simulink model "sampleModel355"  (R2021b)
settings: Solver=VariableStepAuto  StartTime=0.0  StopTime=10.0  RelTol=1e-3
undefined symbols (not defined in the file or in its folder): Newton, Raphson
libraries: simulink x9, slpidlib x1
settings Model: Creator=user  LastModifiedBy=user

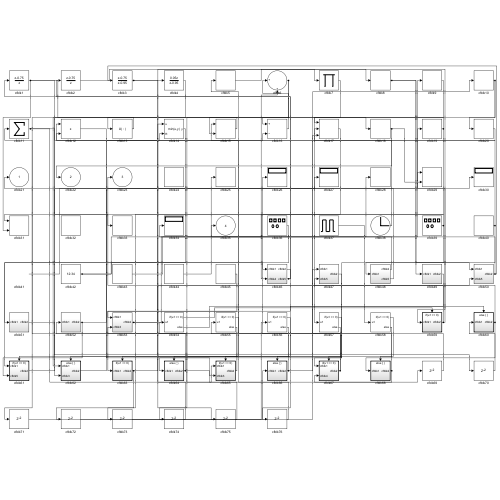
[thumbnail: Simulink's stored preview of the top-level diagram]
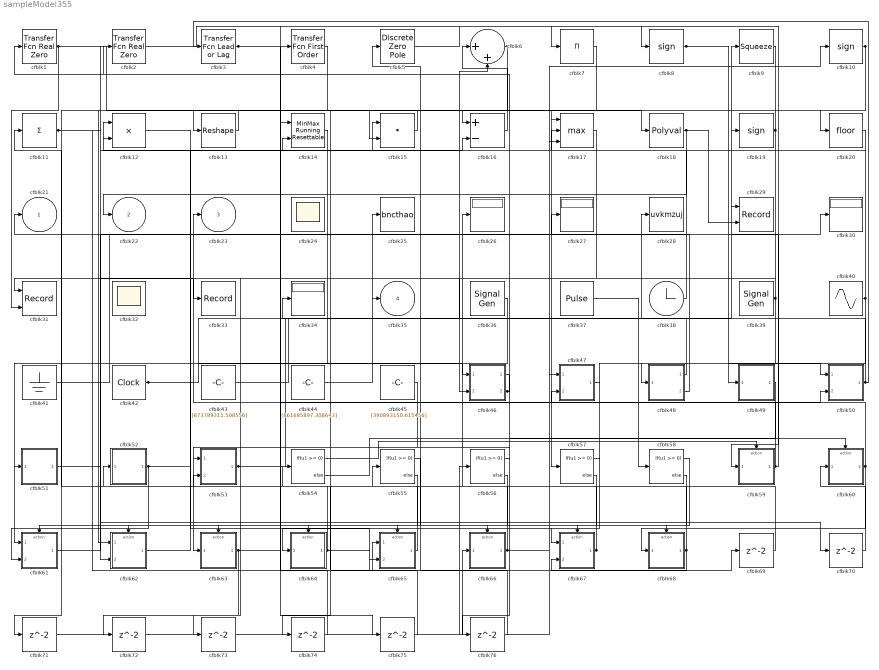
== system sampleModel355 ==
  cfblk1 : simulink/Discrete/Transfer Fcn Real Zero  ZeroZ=0.75  ICPrevInput=0.0  DoSatur=off
      settings: SourceProductBaseCode=SL
  cfblk10 : Signum
  cfblk11 : Sum  Inputs=+
  cfblk12 : Product
  cfblk13 : Reshape
  cfblk14 : simulink/Math Operations/MinMax Running Resettable  Function=min  vinit=0.0
  cfblk15 : DotProduct  InputSameDT=on  OutDataTypeStr=Inherit: Inherit via internal rule
  cfblk16 : Sum  Inputs=+-
  cfblk17 : MinMax  Function=max  Inputs=3
  cfblk18 : Polyval  Coefs=[ +2.081618890e-019, -1.441693666e-014, +4.719686976e-010, -8.536869453e-006, +1.621573104e-001, -8.087801117e+001 ]
  cfblk19 : Signum
  cfblk2 : simulink/Discrete/Transfer Fcn Real Zero  ZeroZ=0.75  ICPrevInput=0.0  DoSatur=off
      settings: SourceProductBaseCode=SL
  cfblk20 : Rounding
  cfblk24 : Scope
      settings: Floating=on
  cfblk25 : ToWorkspace  VariableName=bncthao  SaveFormat=Timeseries  SampleTime=-1
  cfblk{26..27,30,34} (4 alike) : Display
  cfblk28 : ToWorkspace  VariableName=uvkmzuj  SaveFormat=Timeseries  SampleTime=-1
  cfblk29 : Record  FileSettingsInternal="{\"entries\":[{\"content\":{\"excelSettings\":{\"content\":{},\"type\":\"Streamout.ExcelSettings\"}},\"type\":\"Streamout.FileSettingStorage\",\"uuid\":\"8a58f875-e99c-4c1f-ba3d-aacceb243502\"}],\"packageUris\":[\"http://schema.mathworks.com/mf0/streamout_blocks/R2020a\"],\"version\":\"1.0\"}"  Layout=[1 1]  SignalsInternal="{\"entries\":[{\"content\":{\"signals\":[{\"content\":{\"blockPath\":[\"sampleModel355/cfblk29\"],\"channel\":[],\"dimensions\":[1],\"domain\":\"sampleModel355/cfblk29\",\"lineColor\":\"#a2142f\",\"plots\":[1],\"port\":1,\"sid\":[\"\"],\"signalID\":14784,\"signalName\":\"cfblk59\"},\"type\":\"RecordBlkView.Signal\",\"uuid\":\"3281cb25-1353-4514-a61d-ab6e319669d4\"},{\"content\":{\"blockPath\":[\"sampleModel355/cfblk29\"],\"channel\":[],\"dimensions\":[1],\"domain\":\"sampleModel355/cfblk29\",\"lineColor\":\"#139fff\",\"plots\":[1],\"port\":2,\"sid\":[\"\"],\"signalID\":14788,\"signalName\":\"cfblk18\"},\"type\":\"RecordBlkView.Signal\",\"uuid\":\"1768254f-e474-4347-aa62-2856f5bec4c9\"}]},\"type\":\"RecordBlkView.InputSignals\",\"uuid\":\"2a2635e2-e26a-4ce4-9f08-0e49d7d24d48\"}],\"packageUris\":[\"http://schema.mathworks.com/mf0/streamout_blocks/R2020a\"],\"version\":\"1.0\"}"  VisualizationBindings="{\"xyplotplugin\":{\"info\":[{\"series\":[{\"bindingParametersList\":[{\"parameter\":\"X-Axis\",\"signalID\":14784,\"signalName\":\"cfblk59\"},{\"parameter\":\"Y-Axis\",\"signalID\":14788,\"signalName\":\"cfblk18\"}],\"seriesID\":4821}],\"subplotID\":1}]}}"  CompatibilityTag=XY
  cfblk3 : simulink/Discrete/Transfer Fcn Lead or Lag  PoleZ=0.95  ZeroZ=0.75  ICPrevOutput=0.0  ICPrevInput=0.0  DoSatur=off
      settings: SourceProductBaseCode=SL
  cfblk31 : Record  FileSettingsInternal="{\"entries\":[{\"content\":{\"excelSettings\":{\"content\":{},\"type\":\"Streamout.ExcelSettings\"}},\"type\":\"Streamout.FileSettingStorage\",\"uuid\":\"e0b827af-2ce3-47de-8a80-2d3021881471\"}],\"packageUris\":[\"http://schema.mathworks.com/mf0/streamout_blocks/R2020a\"],\"version\":\"1.0\"}"  Layout=[1 1]  SignalsInternal="{\"entries\":[{\"content\":{\"signals\":[{\"content\":{\"blockPath\":[\"sampleModel355/cfblk31\"],\"channel\":[],\"dimensions\":[1],\"domain\":\"sampleModel355/cfblk31\",\"lineColor\":\"#a2142f\",\"plots\":[1],\"port\":1,\"sid\":[\"\"],\"signalID\":14792,\"signalName\":\"cfblk39\"},\"type\":\"RecordBlkView.Signal\",\"uuid\":\"d5c8587e-9d0d-4856-a276-2f59d04580e3\"},{\"content\":{\"blockPath\":[\"sampleModel355/cfblk31\"],\"channel\":[],\"dimensions\":[1],\"domain\":\"sampleModel355/cfblk31\",\"lineColor\":\"#139fff\",\"plots\":[1],\"port\":2,\"sid\":[\"\"],\"signalID\":14796,\"signalName\":\"cfblk1\"},\"type\":\"RecordBlkView.Signal\",\"uuid\":\"aa1322fa-e07b-483b-ac97-480c34133d89\"}]},\"type\":\"RecordBlkView.InputSignals\",\"uuid\":\"07742f17-6200-4858-a083-7661228713f7\"}],\"packageUris\":[\"http://schema.mathworks.com/mf0/streamout_blocks/R2020a\"],\"version\":\"1.0\"}"  VisualizationBindings="{\"xyplotplugin\":{\"info\":[{\"series\":[{\"bindingParametersList\":[{\"parameter\":\"X-Axis\",\"signalID\":14792,\"signalName\":\"cfblk39\"},{\"parameter\":\"Y-Axis\",\"signalID\":14796,\"signalName\":\"cfblk1\"}],\"seriesID\":38022}],\"subplotID\":1}]}}"  CompatibilityTag=XY
  cfblk32 : Scope
      settings: Floating=on
  cfblk33 : Record  FileSettingsInternal="{\"entries\":[{\"content\":{\"excelSettings\":{\"content\":{},\"type\":\"Streamout.ExcelSettings\"}},\"type\":\"Streamout.FileSettingStorage\",\"uuid\":\"c00efc17-803b-4ade-8a07-207905a6f958\"}],\"packageUris\":[\"http://schema.mathworks.com/mf0/streamout_blocks/R2020a\"],\"version\":\"1.0\"}"  SignalsInternal="{\"entries\":[{\"content\":{\"signals\":[{\"content\":{\"blockPath\":[\"sampleModel355/cfblk33\"],\"channel\":[],\"dimensions\":[1],\"domain\":\"sampleModel355/cfblk33\",\"lineColor\":\"#ff6929\",\"plots\":[1],\"port\":1,\"sid\":[\"\"],\"signalID\":14800,\"signalName\":\"cfblk1\"},\"type\":\"RecordBlkView.Signal\",\"uuid\":\"a33f1148-dedf-40b2-8a89-151bff7921ef\"}]},\"type\":\"RecordBlkView.InputSignals\",\"uuid\":\"1131e995-cc5f-4030-b347-0cd77ca9cc44\"}],\"packageUris\":[\"http://schema.mathworks.com/mf0/streamout_blocks/R2020a\"],\"version\":\"1.0\"}"  VisualizationBindings="{\"sparklinesplugin\":{\"info\":[{\"bindingParametersList\":[],\"subplotID\":1}]}}"
  cfblk36 : SignalGenerator  WaveForm=square  Amplitude=[571784640.695162]
  cfblk37 : DiscretePulseGenerator  PulseType=Time based  Amplitude=[-715722832.893154]  Period=[69656277.963047]  PulseWidth=5  PhaseDelay=[1.000000]
  cfblk38 : Clock
  cfblk39 : SignalGenerator  WaveForm=sawtooth  Amplitude=[736063018.120094]
  cfblk4 : simulink/Discrete/Transfer Fcn First Order  PoleZ=0.95  ICPrevOutput=0.0  DoSatur=off
  cfblk40 : Sin  Amplitude=[16568811.325818]  Bias=[-756437996.866727]  SampleTime=0
  cfblk41 : Ground
  cfblk42 : DigitalClock
  cfblk43 : Constant  Value=[873789311.508556]  SampleTime=1
  cfblk44 : Constant  Value=[861685897.308643]  SampleTime=1
  cfblk45 : Constant  Value=[390893150.615456]  SampleTime=1
  cfblk46 : Subsystem
  cfblk47 : Subsystem
  cfblk48 : Subsystem
  cfblk49 : Subsystem
  cfblk5 : DiscreteZeroPole  Poles=[0 0.5]  Gain=1
  cfblk50 : Subsystem
  cfblk51 : Subsystem
  cfblk52 : Subsystem
  cfblk53 : Subsystem
  cfblk{54..58} (5 alike) : If  IfExpression=u1 >= 0  SampleTime=1
  cfblk59 : Subsystem  TreatAsAtomicUnit=on
  cfblk6 : Sum  Inputs=|++
  cfblk60 : Subsystem  TreatAsAtomicUnit=on
  cfblk61 : Subsystem  TreatAsAtomicUnit=on
  cfblk62 : Subsystem  TreatAsAtomicUnit=on
  cfblk63 : Subsystem  TreatAsAtomicUnit=on
  cfblk64 : Subsystem  TreatAsAtomicUnit=on
  cfblk65 : Subsystem  TreatAsAtomicUnit=on
  cfblk66 : Subsystem  TreatAsAtomicUnit=on
  cfblk67 : Subsystem  TreatAsAtomicUnit=on
  cfblk68 : Subsystem  TreatAsAtomicUnit=on
  cfblk{69..76} (8 alike) : Delay  SampleTime=1
  cfblk7 : Product  Inputs=*
  cfblk8 : Signum
  cfblk9 : Squeeze
  cfblk21 : Outport
  cfblk22 : Outport  Port=2
  cfblk23 : Outport  Port=3
  cfblk35 : Outport  Port=4
  wires:
  cfblk9/1 -> cfblk57/1
  cfblk47/1(cfblk2) -> cfblk64/1(cfblk1)
  cfblk68/1(cfblk2) -> cfblk55/1, cfblk67/2(cfblk4)
  cfblk38/1 -> cfblk12/1
  cfblk2/1 -> cfblk59/1(cfblk1)
  cfblk63/1(cfblk2) -> cfblk4/1, cfblk72/1
  cfblk13/1 -> cfblk62/1(cfblk1)
  cfblk11/1 -> cfblk65/1(cfblk1), cfblk16/2
  cfblk64/1(cfblk2) -> cfblk11/1, cfblk69/1
  cfblk61/1(cfblk2) -> cfblk27/1
  cfblk18/1 -> cfblk22/1, cfblk29/2
  cfblk36/1 -> cfblk61/1(cfblk1)
  cfblk59/1(cfblk2) -> cfblk47/2(cfblk5), cfblk29/1
  cfblk10/1 -> cfblk20/1, cfblk74/1
  cfblk16/1 -> cfblk6/1
  cfblk52/1(cfblk2) -> cfblk61/2(cfblk5), cfblk14/2
  cfblk19/1 -> cfblk17/1, cfblk46/2(cfblk4)
  cfblk48/1(cfblk2) -> cfblk34/1
  cfblk65/1(cfblk2) -> cfblk52/1(cfblk1)
  cfblk4/1 -> cfblk62/2(cfblk3)
  cfblk66/1(cfblk2) -> cfblk26/1, cfblk10/1
  cfblk3/1 -> cfblk7/1, cfblk75/1
  cfblk45/1 -> cfblk63/1(cfblk1)
  cfblk41/1 -> cfblk9/1
  cfblk15/1 -> cfblk13/1
  cfblk62/1(cfblk2) -> cfblk30/1
  cfblk42/1 -> cfblk6/2, cfblk46/1(cfblk1)
  cfblk46/1(cfblk2) -> cfblk53/1(cfblk1)
  cfblk43/1 -> cfblk19/1
  cfblk8/1 -> cfblk49/1(cfblk1), cfblk50/1(cfblk1)
  cfblk53/1(cfblk2) -> cfblk28/1, cfblk50/2(cfblk5)
  cfblk40/1 -> cfblk48/1(cfblk1), cfblk12/2
  cfblk48/2(cfblk5) -> cfblk21/1
  cfblk5/1 -> cfblk8/1
  cfblk12/1 -> cfblk65/2(cfblk3)
  cfblk44/1 -> cfblk25/1
  cfblk50/1(cfblk2) -> cfblk3/1, cfblk35/1
  cfblk14/1 -> cfblk51/1(cfblk1)
  cfblk60/1(cfblk2) -> cfblk23/1, cfblk68/1(cfblk1)
  cfblk7/1 -> cfblk16/1
  cfblk20/1 -> cfblk17/2
  cfblk67/1(cfblk2) -> cfblk53/2(cfblk3), cfblk15/1
  cfblk39/1 -> cfblk67/1(cfblk1), cfblk31/1
  cfblk1/1 -> cfblk18/1, cfblk33/1, cfblk31/2
  cfblk37/1 -> cfblk58/1
  cfblk46/2(cfblk5) -> cfblk2/1, cfblk1/1
  cfblk6/1 -> cfblk15/2, cfblk71/1
  cfblk54/1 -> cfblk59/Action
  cfblk54/2 -> cfblk60/Action
  cfblk55/1 -> cfblk61/Action
  cfblk55/2 -> cfblk62/Action
  cfblk56/1 -> cfblk63/Action
  cfblk56/2 -> cfblk64/Action
  cfblk57/1 -> cfblk65/Action
  cfblk57/2 -> cfblk66/Action
  cfblk58/1 -> cfblk67/Action
  cfblk58/2 -> cfblk68/Action
  cfblk69/1 -> cfblk47/1(cfblk1)
  cfblk51/1(cfblk2) -> cfblk70/1
  cfblk70/1 -> cfblk60/1(cfblk1)
  cfblk71/1 -> cfblk66/1(cfblk1)
  cfblk72/1 -> cfblk17/3
  cfblk17/1 -> cfblk73/1
  cfblk73/1 -> cfblk56/1
  cfblk74/1 -> cfblk14/1
  cfblk75/1 -> cfblk54/1
  cfblk49/1(cfblk2) -> cfblk76/1
  cfblk76/1 -> cfblk5/1

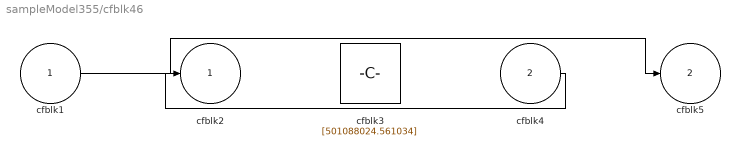
== system sampleModel355/cfblk46 ==
  cfblk1 : Inport
  cfblk4 : Inport  Port=2
  cfblk3 : Constant  Value=[501088024.561034]  SampleTime=1
  cfblk2 : Outport
  cfblk5 : Outport  Port=2
  wires:
  cfblk1/1 -> cfblk5/1
  cfblk4/1 -> cfblk2/1

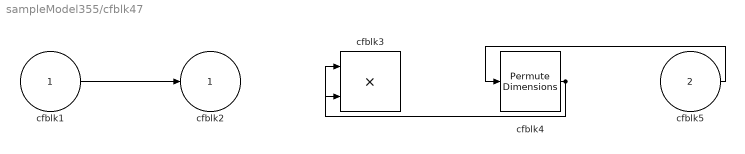
== system sampleModel355/cfblk47 ==
  cfblk1 : Inport
  cfblk5 : Inport  Port=2
  cfblk3 : Product  Inputs=**
  cfblk4 : PermuteDimensions
  cfblk2 : Outport
  wires:
  cfblk5/1 -> cfblk4/1
  cfblk1/1 -> cfblk2/1
  cfblk4/1 -> cfblk3/1, cfblk3/2

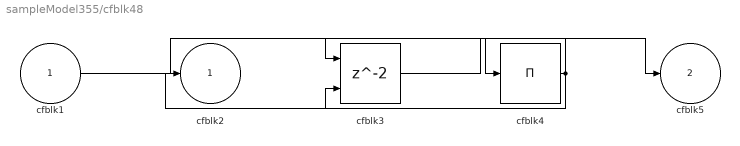
== system sampleModel355/cfblk48 ==
  cfblk1 : Inport
  cfblk3 : Delay  ShowEnablePort=on  SampleTime=1
      settings: InputPortMap=u0,e6
  cfblk4 : Product  Inputs=*
  cfblk2 : Outport
  cfblk5 : Outport  Port=2
  wires:
  cfblk1/1 -> cfblk4/1
  cfblk4/1 -> cfblk2/1, cfblk3/1, cfblk3/2
  cfblk3/1 -> cfblk5/1

== system sampleModel355/cfblk49 ==
  cfblk1 : Inport
  cfblk3 : Sqrt  Operator=rSqrt  AlgorithmType=Newton-Raphson  SaturateOnIntegerOverflow=on
  cfblk2 : Outport
  wires:
  cfblk3/1 -> cfblk2/1
  cfblk1/1 -> cfblk3/1

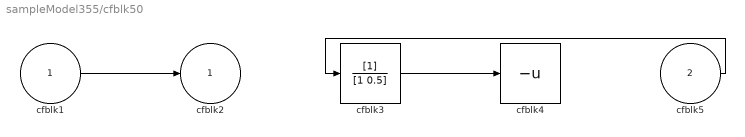
== system sampleModel355/cfblk50 ==
  cfblk1 : Inport
  cfblk5 : Inport  Port=2
  cfblk3 : DiscreteFilter  SampleTime=1
  cfblk4 : UnaryMinus
  cfblk2 : Outport
  wires:
  cfblk1/1 -> cfblk2/1
  cfblk3/1 -> cfblk4/1
  cfblk5/1 -> cfblk3/1

== system sampleModel355/cfblk51 ==
  cfblk1 : Inport
  cfblk3 : DiscreteZeroPole  Poles=[0 0.5]  Gain=1
  cfblk2 : Outport
  wires:
  cfblk1/1 -> cfblk3/1
  cfblk3/1 -> cfblk2/1

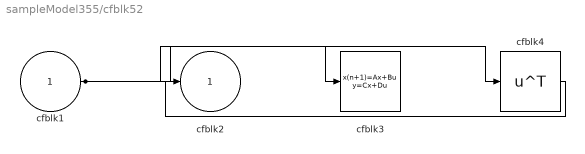
== system sampleModel355/cfblk52 ==
  cfblk1 : Inport
  cfblk3 : DiscreteStateSpace
  cfblk4 : Math  Operator=transpose  SaturateOnIntegerOverflow=on
  cfblk2 : Outport
  wires:
  cfblk1/1 -> cfblk4/1, cfblk3/1
  cfblk4/1 -> cfblk2/1

== system sampleModel355/cfblk53 ==
  cfblk1 : Inport
  cfblk3 : Inport  Port=2
  cfblk2 : Outport
  wires:
  cfblk1/1 -> cfblk2/1

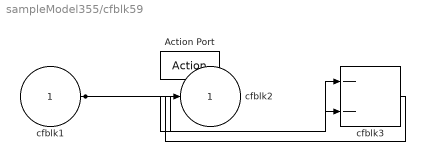
== system sampleModel355/cfblk59 ==
  cfblk1 : Inport
  Action Port : ActionPort  ActionPortLabel=if(u1 >= 0)
  cfblk3 : Sum  Inputs=--
  cfblk2 : Outport
  wires:
  cfblk1/1 -> cfblk3/1, cfblk3/2
  cfblk3/1 -> cfblk2/1

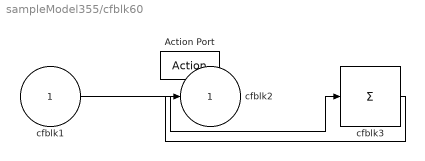
== system sampleModel355/cfblk60 ==
  cfblk1 : Inport
  Action Port : ActionPort  ActionPortLabel=else
  cfblk3 : Sum  Inputs=+
  cfblk2 : Outport
  wires:
  cfblk1/1 -> cfblk3/1
  cfblk3/1 -> cfblk2/1

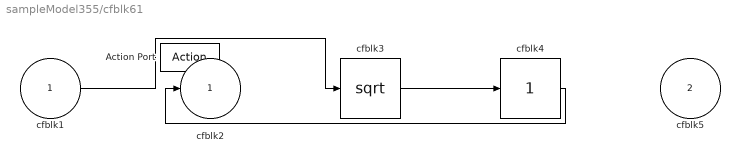
== system sampleModel355/cfblk61 ==
  cfblk1 : Inport
  cfblk5 : Inport  Port=2
  Action Port : ActionPort  ActionPortLabel=if(u1 >= 0)
  cfblk3 : Sqrt  SaturateOnIntegerOverflow=on
  cfblk4 : simulink/Math Operations/Slider Gain  gain=1  low=0  high=2
  cfblk2 : Outport
  wires:
  cfblk4/1 -> cfblk2/1
  cfblk3/1 -> cfblk4/1
  cfblk1/1 -> cfblk3/1

== system sampleModel355/cfblk62 ==
  cfblk1 : Inport
  cfblk3 : Inport  Port=2
  Action Port : ActionPort  ActionPortLabel=else
  cfblk2 : Outport
  wires:
  cfblk1/1 -> cfblk2/1

== system sampleModel355/cfblk63 ==
  cfblk1 : Inport
  Action Port : ActionPort  ActionPortLabel=if(u1 >= 0)
  cfblk3 : DotProduct  InputSameDT=on  OutDataTypeStr=Inherit: Inherit via internal rule
  cfblk2 : Outport
  wires:
  cfblk3/1 -> cfblk2/1
  cfblk1/1 -> cfblk3/1, cfblk3/2

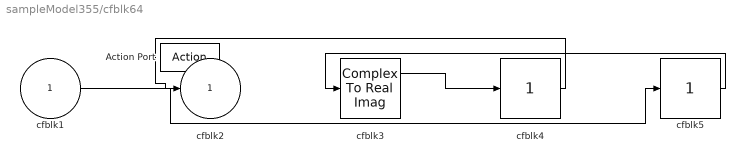
== system sampleModel355/cfblk64 ==
  cfblk1 : Inport
  Action Port : ActionPort  ActionPortLabel=else
  cfblk3 : ComplexToRealImag
  cfblk4 : simulink/Math Operations/Slider Gain  gain=1  low=0  high=2
  cfblk5 : simulink/Math Operations/Slider Gain  gain=1  low=0  high=2
  cfblk2 : Outport
  wires:
  cfblk1/1 -> cfblk5/1
  cfblk4/1 -> cfblk2/1
  cfblk5/1 -> cfblk3/1
  cfblk3/1 -> cfblk4/1

== system sampleModel355/cfblk65 ==
  cfblk1 : Inport
  cfblk3 : Inport  Port=2
  Action Port : ActionPort  ActionPortLabel=if(u1 >= 0)
  cfblk2 : Outport
  wires:
  cfblk3/1 -> cfblk2/1

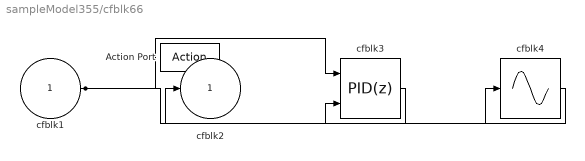
== system sampleModel355/cfblk66 ==
  cfblk1 : Inport
  Action Port : ActionPort  ActionPortLabel=else
  cfblk3 : slpidlib/PID Controller (2DOF)  Controller=PID  Form=Parallel  TimeDomain=Discrete-time  UseExternalTs=off  SampleTime=-1  IntegratorMethod=Forward Euler  FilterMethod=Forward Euler  ControllerParametersSource=internal  P=1  I=1  D=0  UseFilter=on  N=100  b=1  c=1  TunerSelectOption=Transfer Function Based (PID Tuner App)  InitialConditionSource=internal  InitialConditionForIntegrator=0  InitialConditionForFilter=0  DifferentiatorICPrevScaledInput=0  ExternalReset=none  TrackingMode=off  Kt=1  LimitOutput=off  SatLimitsSource=internal  UpperSaturationLimit=inf  LowerSaturationLimit=-inf  LinearizeAsGain=off  AntiWindupMode=none  Kb=1  POutMin=[]  POutMax=[]  IOutMin=[]  IOutMax=[]  DOutMin=[]  DOutMax=[]  NOutMin=[]  NOutMax=[]  bOutMin=[]  bOutMax=[]  cOutMin=[]  cOutMax=[]  SumOutMin=[]  SumOutMax=[]  SaturationOutMin=[]  SaturationOutMax=[]  PParamMin=[]  PParamMax=[]  IParamMin=[]  IParamMax=[]  DParamMin=[]  DParamMax=[]  NParamMin=[]  NParamMax=[]  bParamMin=[]  bParamMax=[]  cParamMin=[]  cParamMax=[]  KbParamMin=[]  KbParamMax=[]  KtParamMin=[]  KtParamMax=[]  KbOutMin=[]  KbOutMax=[]  KtOutMin=[]  KtOutMax=[]  IntegratorOutMin=[]  IntegratorOutMax=[]  FilterOutMin=[]  FilterOutMax=[]  SumI1OutMin=[]  SumI1OutMax=[]  SumI2OutMin=[]  SumI2OutMax=[]  SumI3OutMin=[]  SumI3OutMax=[]  SumI4OutMin=[]  SumI4OutMax=[]  SumDOutMin=[]  SumDOutMax=[]  Sum1OutMin=[]  Sum1OutMax=[]  Sum2OutMin=[]  Sum2OutMax=[]  Sum3OutMin=[]  Sum3OutMax=[]  DifferentiatorOutMin=[]  DifferentiatorOutMax=[]  FilterDiffOutCoefMin=[]  FilterDiffOutCoefMax=[]  ReciprocalOutMin=[]  ReciprocalOutMax=[]  SumDenOutMin=[]  SumDenOutMax=[]  SumNumOutMin=[]  SumNumOutMax=[]  DivideOutMin=[]  DivideOutMax=[]  UdiffTsProdOutMin=[]  UdiffTsProdOutMax=[]  NTsProdOutMin=[]  NTsProdOutMax=[]  UintegralTsProdOutMin=[]  UintegralTsProdOutMax=[]  UngainTsProdOutMin=[]  UngainTsProdOutMax=[]  IntegratorContinuousStateAttributes=''  IntegratorStateMustResolveToSignalObject=off  IntegratorRTWStateStorageClass=Auto  FilterContinuousStateAttributes=''  FilterStateMustResolveToSignalObject=off  FilterRTWStateStorageClass=Auto  ParallelPVariant=InternalParameters  IdealPVariant=Disabled  IVariant=InternalParameters  DVariant=InternalParameters  bVariant=InternalParameters  cVariant=InternalParameters  IntegratorVariant=Discrete  SatVariant=Disabled  AWVariant=Passthrough  PCopyVariant=Disabled  TRVariant=Disabled  FdbkBlocksVariant=Forward  IdealPFdbkVariant=Disabled  SatFdbkVariant=Disabled  DerivativeFilterVariant=ForwardEulerFilter  NVariant=InternalParameters  NCopyVariant=Disabled  FilterICVariant=InternalICsFilter  IntegratorICVariant=InternalICs  ExternalResetVariant=Disabled  TRSumVariant=Passthrough  SumFdbkVariant=Disabled  SumVariant=Sum_PID  TsampFilterVariant=InternalTs  TsampNgainVariant=Passthrough  TsampIntegralVariant=Passthrough  ExternalSaturationOutDataTypeStr=Inherit: Same as second input
      settings: SourceProductBaseCode=SL
  cfblk4 : Sin  TimeSource=Use external signal  SampleTime=0
  cfblk2 : Outport
  wires:
  cfblk3/1 -> cfblk2/1
  cfblk1/1 -> cfblk3/1, cfblk4/1
  cfblk4/1 -> cfblk3/2

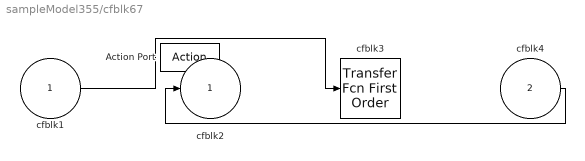
== system sampleModel355/cfblk67 ==
  cfblk1 : Inport
  cfblk4 : Inport  Port=2
  Action Port : ActionPort  ActionPortLabel=if(u1 >= 0)
  cfblk3 : simulink/Discrete/Transfer Fcn First Order  PoleZ=0.95  ICPrevOutput=0.0  DoSatur=off
  cfblk2 : Outport
  wires:
  cfblk4/1 -> cfblk2/1
  cfblk1/1 -> cfblk3/1

== system sampleModel355/cfblk68 ==
  cfblk1 : Inport
  Action Port : ActionPort  ActionPortLabel=else
  cfblk3 : Math  Operator=log  SaturateOnIntegerOverflow=on
  cfblk2 : Outport
  wires:
  cfblk3/1 -> cfblk2/1
  cfblk1/1 -> cfblk3/1
